simulink model "SMCmarine"  (R2018b)
settings: Solver=FixedStepAuto  StartTime=0.0  StopTime=600  FixedStep=0.06  RelTol=1e-3
libraries: simulink x1
settings Model: Creator=User  LastModifiedBy=User

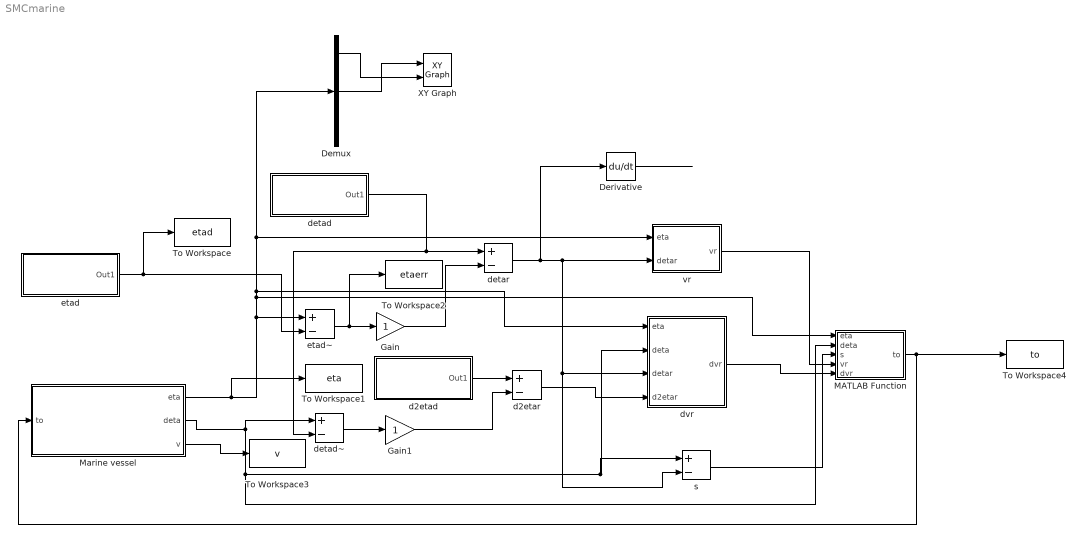
== system SMCmarine ==
  Demux : Demux  Outputs=3
  Derivative : Derivative
  Gain : Gain
  Gain1 : Gain
  MATLAB Function : MATLAB Function  TreatAsAtomicUnit=on
  Marine vessel : Subsystem
  To Workspace : ToWorkspace  VariableName=etad  SampleTime=-1
  To Workspace1 : ToWorkspace  VariableName=eta  SampleTime=-1
  To Workspace2 : ToWorkspace  VariableName=etaerr  SampleTime=-1
  To Workspace3 : ToWorkspace  VariableName=v  SampleTime=-1
  To Workspace4 : ToWorkspace  VariableName=to  SampleTime=-1
  XY Graph : simulink/Sinks/XY Graph  xmin=-3000  xmax=3000  ymin=-3000  ymax=3000  st=-1
  d2etad : Subsystem
  d2etar : Sum  Inputs=+-
  detad : Subsystem
  detad~ : Sum  Inputs=+-
  detar : Sum  Inputs=+-
  dvr : MATLAB Function  TreatAsAtomicUnit=on
  etad : Subsystem
  etad~ : Sum  Inputs=+-
  s : Sum  Inputs=+-
  vr : MATLAB Function  TreatAsAtomicUnit=on
  wires:
  Marine vessel/1(eta) -> To Workspace1/1, Demux/1, vr/1(eta), dvr/1(eta), MATLAB Function/1(eta), etad~/1
  etad/1(Out1) -> To Workspace/1, etad~/2
  detad/1(Out1) -> detad~/2, detar/1
  etad~/1 -> To Workspace2/1, Gain/1
  Gain/1 -> detar/2
  d2etad/1(Out1) -> d2etar/1
  Marine vessel/2(deta) -> MATLAB Function/2(deta), s/1, dvr/2(deta), detad~/1
  Gain1/1 -> d2etar/2
  detar/1 -> Derivative/1, s/2, dvr/3(detar), vr/2(detar)
  d2etar/1 -> dvr/4(d2etar)
  dvr/1(dvr) -> MATLAB Function/5(dvr)
  vr/1(vr) -> MATLAB Function/4(vr)
  s/1 -> MATLAB Function/3(s)
  MATLAB Function/1(to) -> Marine vessel/1(to), To Workspace4/1
  Derivative/1 -> ?
  detad~/1 -> Gain1/1
  Demux/2 -> XY Graph/1
  Demux/1 -> XY Graph/2
  Marine vessel/3(v) -> To Workspace3/1

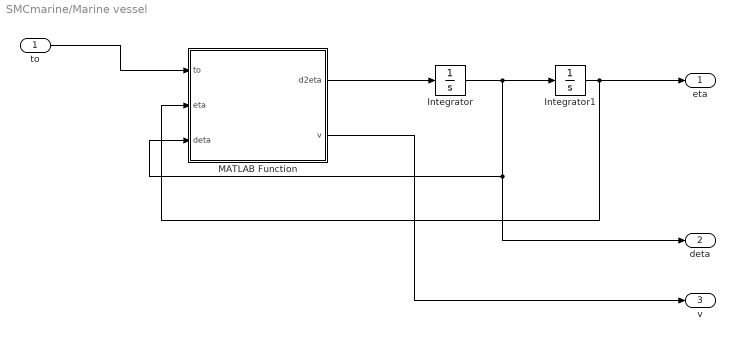
== system SMCmarine/Marine vessel ==
  to : Inport
  Integrator : Integrator  InitialCondition=[0;0;0]
  Integrator1 : Integrator  InitialCondition=[-100;800;pi/2]
  MATLAB Function : MATLAB Function  TreatAsAtomicUnit=on
  eta : Outport
  deta : Outport  Port=2
  v : Outport  Port=3
  wires:
  Integrator1/1 -> eta/1, MATLAB Function/2(eta)
  MATLAB Function/1(d2eta) -> Integrator/1
  Integrator/1 -> deta/1, MATLAB Function/3(deta), Integrator1/1
  to/1 -> MATLAB Function/1(to)
  MATLAB Function/2(v) -> v/1

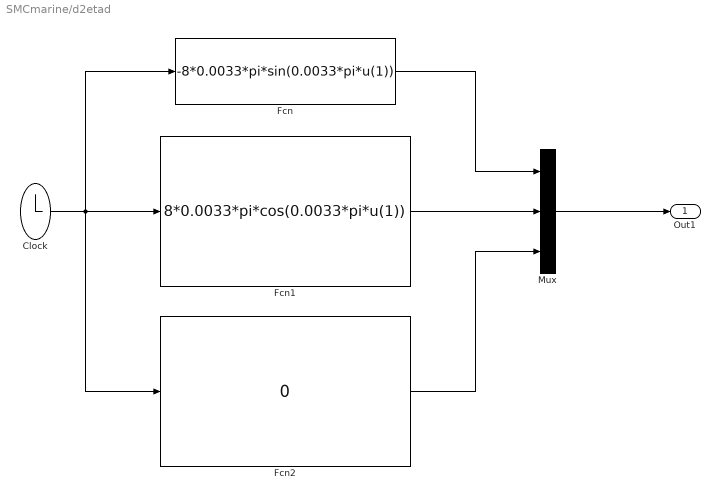
== system SMCmarine/d2etad ==
  Clock : Clock
  Fcn : Fcn  Expr=-8*0.0033*pi*sin(0.0033*pi*u(1))
  Fcn1 : Fcn  Expr=8*0.0033*pi*cos(0.0033*pi*u(1))
  Fcn2 : Fcn  Expr=0
  Mux : Mux  Inputs=3
  Out1 : Outport
  wires:
  Clock/1 -> Fcn2/1, Fcn/1, Fcn1/1
  Fcn/1 -> Mux/1
  Fcn1/1 -> Mux/2
  Fcn2/1 -> Mux/3
  Mux/1 -> Out1/1

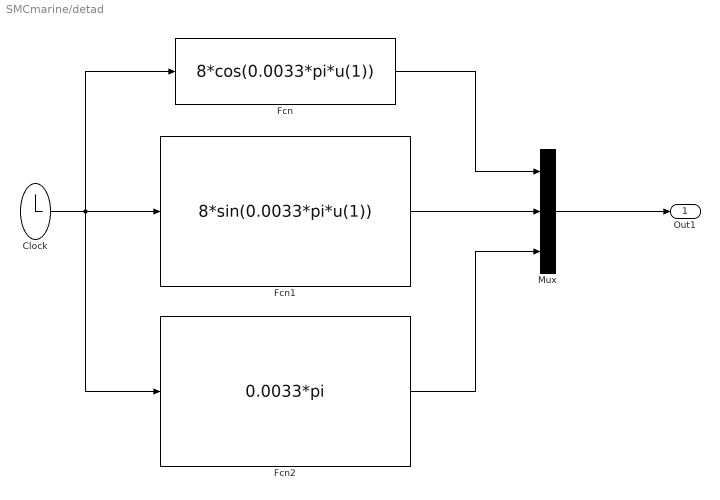
== system SMCmarine/detad ==
  Clock : Clock
  Fcn : Fcn  Expr=8*cos(0.0033*pi*u(1))
  Fcn1 : Fcn  Expr=8*sin(0.0033*pi*u(1))
  Fcn2 : Fcn  Expr=0.0033*pi
  Mux : Mux  Inputs=3
  Out1 : Outport
  wires:
  Mux/1 -> Out1/1
  Fcn2/1 -> Mux/3
  Fcn1/1 -> Mux/2
  Fcn/1 -> Mux/1
  Clock/1 -> Fcn1/1, Fcn/1, Fcn2/1

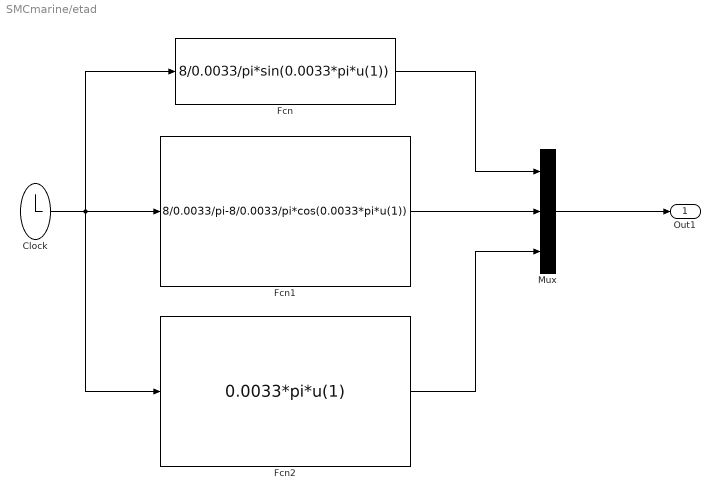
== system SMCmarine/etad ==
  Clock : Clock
  Fcn : Fcn  Expr=8/0.0033/pi*sin(0.0033*pi*u(1))
  Fcn1 : Fcn  Expr=8/0.0033/pi-8/0.0033/pi*cos(0.0033*pi*u(1))
  Fcn2 : Fcn  Expr=0.0033*pi*u(1)
  Mux : Mux  Inputs=3
  Out1 : Outport
  wires:
  Clock/1 -> Fcn2/1, Fcn/1, Fcn1/1
  Fcn/1 -> Mux/1
  Fcn1/1 -> Mux/2
  Fcn2/1 -> Mux/3
  Mux/1 -> Out1/1

== matlab function SMCmarine/vr ==
  data: eta input; vr output; detar input
function vr = fcn(eta,detar)
J=[cos(eta(3)) -sin(eta(3)) 0;
    sin(eta(3)) cos(eta(3)) 0;
    0 0 1];
vr=J'*detar;
end

== matlab function SMCmarine/Marine vessel/MATLAB Function ==
  data: d2eta output; to input; eta input; deta input; v output
function [d2eta,v] = fcn(to,eta,deta)
J=[cos(eta(3)) -sin(eta(3)) 0;
    sin(eta(3)) cos(eta(3)) 0;
    0 0 1];
v=J'*deta;
M=1e6*[4.5096 0 0;0 7.5608 -22.68;0 -22.68 2968.3];
c13=-7.5608*v(2)+22.68*v(3);
c23=4.5096*v(1);
c31=-c13;
c32=-c23;
C=[0 0 c13;0 0 c23;c31 c32 0];
D=1e6*[0.05138 0 0;0 0.1698 -1.5081;0 -1.5081 253];
S=[0 -deta(3) 0;
    deta(3) 0 0;
    0 0 0];
Meta=M*J';
Ceta=(C-M*S)*J';
Deta=D*J';
d2eta=Meta\(to-Ceta*deta-Deta*deta);
end

== matlab function SMCmarine/dvr ==
  data: eta input; deta input; dvr output; detar input; d2etar input
function dvr = fcn(eta,deta,detar,d2etar)
J=[cos(eta(3)) -sin(eta(3)) 0;
    sin(eta(3)) cos(eta(3)) 0;
    0 0 1];
S=[0 -deta(3) 0;
    deta(3) 0 0;
    0 0 0];
dvr=-S*J'*detar+J'*d2etar;
end

== matlab function SMCmarine/MATLAB Function ==
  data: eta input; to output; deta input; s input; vr input; dvr input
function to = fcn(eta,deta,s,vr,dvr)
J=[cos(eta(3)) -sin(eta(3)) 0;
    sin(eta(3)) cos(eta(3)) 0;
    0 0 1];
v=J'*deta;
M=1e6*[4.5096 0 0;0 7.5608 -22.68;0 -22.68 2968.3];
c13=-7.5608*v(2)+22.68*v(3);
c23=4.5096*v(1);
c31=-c13;
c32=-c23;
C=[0 0 c13;0 0 c23;c31 c32 0];
D=1e6*[0.05138 0 0;0 0.1698 -1.5081;0 -1.5081 253];
S=[0 -deta(3) 0;
    deta(3) 0 0;
    0 0 0];
Meta=M*J';
Ceta=(C-M*S)*J';
Deta=D*J';
to=M*dvr+C*vr+D*vr+(Ceta+Deta)*s-Meta*(diag([1 2 8]*1e-2)*s+1e-2*sign(s));
end
